simulink model "TVModel_Simulation"  (R2022a)
settings: Solver=FixedStepDiscrete  StartTime=0.0  StopTime=200  FixedStep=0.02  MaxStep=0.01  RelTol=1e-3
undefined symbols (not defined in the file or in its folder): TV
libraries: simulink x5, simulink_extras x3, dspstat3 x2, sharedTrackingLibrary x1, slpidlib x1, eeGeneralControl x1
(part 3 of 4)

== system TVModel_Simulation/Subsystem/Subsystem1/Torque Distribution/MPC/Faults detection/Subsystem2 ==
  In Bus Element : Inport  PortName=dynamics_data  Element=vx
  In Bus Element1 : Inport  Port=2  PortName=driver_inputs  Element=throttle
  OCP Status : Inport  Port=3
  Constant : Constant  Value=3
  Constant1 : Constant  Value=TV.MPC.N/TV.MPC.T*0.1-1
  Constant2 : Constant  Value=TV.LV.TORQUE.T_peak_motor*[0.3;0.3;1;1]
  Discrete FIR Filter : DiscreteFir  Coefficients=ones(1,TV.MPC.N/TV.MPC.T*0.1)
  Less Than : RelationalOperator  Operator=<  OutDataTypeStr=boolean  RndMeth=Simplest  InputSameDT=off
  Less Than1 : RelationalOperator  OutDataTypeStr=boolean  RndMeth=Simplest  InputSameDT=off
  OR : Logic  Operator=OR  Inputs=1  IconShape=distinctive  AllPortsSameDT=off  OutDataTypeStr=boolean
  Product : Product
  Simple Torque : Outport
  flag : Outport  Port=2
  wires:
  OCP Status/1 -> Discrete FIR Filter/1
  Less Than1/1 -> ?  "buffer_flag"
  Discrete FIR Filter/1 -> Less Than1/1
  Constant1/1 -> Less Than1/2
  Product/1 -> Simple Torque/1
  In Bus Element1/1 -> Product/1
  Constant2/1 -> Product/2
  Less Than/1 -> OR/1, flag/1
  In Bus Element/1 -> Less Than/1  "vx"
  Constant/1 -> Less Than/2

== system TVModel_Simulation/Subsystem/Subsystem1/Torque Distribution/MPC/Polytopic Constraints/Accelerator mapping  ==
  acc : Inport
  Constant : Constant
  Divide : Product  Inputs=*/
  Divide1 : Product  Inputs=/*
  Exponent < 0 : Constant  Value=-1.5
  Power : Math  Operator=pow
  Subtract : Sum  Inputs=-+
  Sum : Sum  Inputs=|++
  mapped acc : Outport
  Out Bus Element1 : Outport  Port=2  PortName=TV_Info  Element=acc_map
  wires:
  acc/1 -> Subtract/1, Divide/1
  Subtract/1 -> Divide/2
  Constant/1 -> Sum/2, Divide1/2, Subtract/2
  Divide/1 -> Power/1
  Exponent < 0/1 -> Power/2
  Power/1 -> Sum/1
  Sum/1 -> Divide1/1
  Divide1/1 -> Out Bus Element1/1, mapped acc/1  "acc_map"

== system TVModel_Simulation/Subsystem/Subsystem1/Torque Distribution/MPC/Polytopic Constraints/Power Limiter ==
  In Bus Element5 : Inport  PortName=hv
  In Bus Element4 : Inport  PortName=hv
  In Bus Element3 : Inport  PortName=hv  Element=Pmax_tractive
  In Bus Element1 : Inport  PortName=hv  Element=current
  In Bus Element2 : Inport  PortName=hv  Element=voltage
  If : If  IfExpression=u1 < 0
  If Action Subsystem : Subsystem  TreatAsAtomicUnit=on
  If Action Subsystem1 : Subsystem  TreatAsAtomicUnit=on
  Merge : Merge
  Product : Product
  Subtract : Sum  Inputs=+-
  Out1 : Outport
  wires:
  In Bus Element1/1 -> Product/1  "hv"
  In Bus Element2/1 -> Product/2  "hv"
  In Bus Element3/1 -> Subtract/1  "hv"
  Product/1 -> Subtract/2
  Subtract/1 -> If Action Subsystem/2(Inport), If/1
  If/1 -> If Action Subsystem/Action
  If/2 -> If Action Subsystem1/Action
  If Action Subsystem1/1(Out1) -> Merge/2
  If Action Subsystem/1(Out1) -> Merge/1
  Merge/1 -> Out1/1
  In Bus Element5/1 -> If Action Subsystem/1(hv)  "hv"
  In Bus Element4/1 -> If Action Subsystem1/1(hv)  "hv"

== system TVModel_Simulation/Subsystem/Subsystem1/Torque Distribution/MPC/Polytropic Matrix/Efficiency limit ==
  Motor_Torque : Inport  OutDataTypeStr=double  PortDimensions=4
  In Bus Element34 : Inport  Port=2  PortName=dynamics_data  Element=omega_wheels
  In Bus Element2 : Inport  Port=2  PortName=dynamics_data  Element=omega_wheels
  "     " : Gain  Gain=TV.LV.inv_efficiency
  "      " : Gain  Gain=1/TV.LV.inv_efficiency
  Constant : Constant
  Divide : Product  Inputs=*/
  Gain2 : Gain  Gain=TV.CAR.Tau
  Power to engines : Subsystem
  Saturation : Saturate  UpperLimit=19900*pi/30  LowerLimit=100*pi/30
  Switch3 : Switch  Criteria=u2 > Threshold  SaturateOnIntegerOverflow=off  InputSameDT=off
  Limit : Outport
  wires:
  Power to engines/1(Efficiency) -> "      "/1, "     "/1
  "      "/1 -> Switch3/3  "Braking"
  "     "/1 -> Switch3/1, Divide/2  "Driving"
  Motor_Torque/1 -> Power to engines/2(Torque)
  In Bus Element34/1 -> Gain2/1
  Gain2/1 -> Saturation/1
  In Bus Element2/1 -> Switch3/2
  Divide/1 -> Limit/1
  Saturation/1 -> Power to engines/1(omega_motor)
  Constant/1 -> Divide/1

== system TVModel_Simulation/Subsystem/Subsystem1/Torque Distribution/MPC/States constraints/Anti reverse wheelspin ==
  lbu_in : Inport
  slip_ratio : Inport  Port=2  PortName=dynamics_data
  Constant : Constant  Value=-0.5
  Less Than : RelationalOperator  OutDataTypeStr=boolean  RndMeth=Simplest  InputSameDT=off
  Product : Product
  lbu_out : Outport
  wires:
  Constant/1 -> Less Than/2
  Less Than/1 -> Product/2
  slip_ratio/1 -> Less Than/1
  lbu_in/1 -> Product/1
  Product/1 -> lbu_out/1  "lbu_out"

== system TVModel_Simulation/Subsystem/Subsystem1/Torque Distribution/MPC/States constraints/Brake & ESP ==
  ubu_in : Inport
  In Bus Element13 : Inport  Port=2  PortName=brake_signal  Element=regen
  Constant : Constant
  Constant1 : Constant  Value=0
  Product : Product
  Switch : Switch  Criteria=u2 > Threshold  Threshold=0.95  SaturateOnIntegerOverflow=off  InputSameDT=off
  ubu_out : Outport
  wires:
  Constant/1 -> Switch/3
  Constant1/1 -> Switch/1
  ubu_in/1 -> Product/1
  Switch/1 -> Product/2
  Product/1 -> ubu_out/1
  In Bus Element13/1 -> Switch/2

== system TVModel_Simulation/Subsystem/Subsystem1/Torque Distribution/MPC/States constraints/Bus lbu ==
  lbu : Inport
  C Function : CFunction  OutputCode=|
      | int i,j;
      | for (i = 0; i < N; i++) {
      |  for (j = 0; j < nu; j++) {
      |   out_x[i*nu+j] = in_x[j];
      |  }
      | }
  Constant1 : Constant  Value=TV.MPC.N-1  OutDataTypeStr=uint8  SampleTime=TV.MPC.T/TV.MPC.N
  Constant3 : Constant  Value=TV.MPC.nu  OutDataTypeStr=uint8  SampleTime=TV.MPC.T/TV.MPC.N
  Out : Outport
  wires:
  Constant1/1 -> C Function/2
  C Function/1 -> Out/1
  Constant3/1 -> C Function/3
  lbu/1 -> C Function/1

== system TVModel_Simulation/Subsystem/Subsystem1/Torque Distribution/MPC/States constraints/Bus ubu ==
  ubu : Inport
  C Function : CFunction  OutputCode=|
      | int i,j;
      | for (i = 0; i < N; i++) {
      |  for (j = 0; j < nu; j++) {
      |   out_x[i*nu+j] = in_x[j];
      |  }
      | }
  Constant1 : Constant  Value=TV.MPC.N-1  OutDataTypeStr=uint8  SampleTime=TV.MPC.T/TV.MPC.N
  Constant3 : Constant  Value=TV.MPC.nu  OutDataTypeStr=uint8  SampleTime=TV.MPC.T/TV.MPC.N
  Out : Outport
  wires:
  Constant1/1 -> C Function/2
  C Function/1 -> Out/1
  Constant3/1 -> C Function/3
  ubu/1 -> C Function/1

== system TVModel_Simulation/Subsystem/Subsystem1/Torque Distribution/MPC/States constraints/Hydraulic brakes ==
  In1 : Inport
  In Bus Element7 : Inport  Port=2  PortName=dynamics_data  Element=brake_torque
  Brake friction : Gain  Commented=on  Gain=0.8
  Braking Areas : Constant  Commented=on  Value=[TV.CAR.BrkArea_front;TV.CAR.BrkArea_front;TV.CAR.BrkArea_rear;TV.CAR.BrkArea_rear]
  Braking Disk Radii : Constant  Commented=on  Value=[TV.CAR.DiskDiameter_front;TV.CAR.DiskDiameter_front;TV.CAR.DiskDiameter_rear;TV.CAR.DiskDiameter_rear]/2
  Product : Product  Commented=on
  Product1 : Product  Commented=on
  Subtract : Sum
  Wheel2Motor : Gain  Gain=1/TV.CAR.Tau
  Out1 : Outport
  wires:
  Brake friction/1 -> Product1/1
  Wheel2Motor/1 -> Subtract/2
  In Bus Element7/1 -> Wheel2Motor/1
  Subtract/1 -> Out1/1
  In1/1 -> Subtract/1
  Braking Areas/1 -> Product/2
  Braking Disk Radii/1 -> Product1/2
  Product/1 -> Brake friction/1

== system TVModel_Simulation/Subsystem/Subsystem1/Torque Distribution/MPC/States constraints/LMUx Correction ==
  LMUx Front : Constant  Value=0.75
  LMUx Rear : Constant  Value=0.75
  Nominal LMUx : Gain  Gain=1/0.93
  Vector Concatenate : Concatenate  NumInputs=4
  Out1 : Outport
  wires:
  LMUx Rear/1 -> Vector Concatenate/4, Vector Concatenate/3
  LMUx Front/1 -> Vector Concatenate/1, Vector Concatenate/2
  Nominal LMUx/1 -> Out1/1
  Vector Concatenate/1 -> Nominal LMUx/1

== system TVModel_Simulation/Subsystem/Subsystem1/Torque Distribution/MPC/States constraints/Load Transfer calculation ==
  In Bus Element : Inport  PortName=dynamics_data
  Fz FL : Subsystem
  Fz FR : Subsystem
  Fz RL : Subsystem
  Fz RR : Subsystem
  Mux : Mux
  Fz [4x1] : Outport
  Out Bus Element4 : Outport  Port=2  PortName=TV_Info  Element=fz_fl
  Out Bus Element1 : Outport  Port=2  PortName=TV_Info  Element=fz_fr
  Out Bus Element2 : Outport  Port=2  PortName=TV_Info  Element=fz_rl
  Out Bus Element3 : Outport  Port=2  PortName=TV_Info  Element=fz_rr
  wires:
  In Bus Element/1 -> Fz FL/1(dynamics_data), Fz FR/1(dynamics_data), Fz RL/1(dynamics_data), Fz RR/1(dynamics_data)
  Fz FL/1(TV_Info) -> Out Bus Element4/1, Mux/1  "Fz_FL"
  Fz FR/1(TV_Info) -> Mux/2, Out Bus Element1/1  "Fz_FR"
  Fz RL/1(TV_Info) -> Out Bus Element2/1, Mux/3  "Fz_RL"
  Fz RR/1(TV_Info) -> Out Bus Element3/1, Mux/4  "Fz_RR"
  Mux/1 -> Fz [4x1]/1

== system TVModel_Simulation/Subsystem/Subsystem1/Torque Distribution/MPC/States constraints/Low YRD ==
  In Bus Element13 : Inport  PortName=brake_signal
  ubu : Inport  Port=2
  YRD : Inport  Port=3
  lbu : Inport  Port=4
  In Bus Element1 : Inport  Port=5  PortName=driver_inputs
  lbu_max : Inport  Port=6
  Demux : Demux
  Demux1 : Demux
  Mux : Mux  Inputs=10
  Mz = 0 Bound logic : Subsystem
  Output : Outport
  wires:
  lbu_max/1 -> Mux/10
  In Bus Element1/1 -> Mz = 0 Bound logic/3(driver_inputs)
  YRD/1 -> Mz = 0 Bound logic/2(YRD)
  In Bus Element13/1 -> Mz = 0 Bound logic/1(brake_signal)
  lbu/1 -> Demux1/1
  Demux1/1 -> Mux/6
  Demux1/4 -> Mux/9
  Demux1/2 -> Mux/7
  Demux1/3 -> Mux/8
  Mz = 0 Bound logic/1(flag) -> Mux/1
  Demux/4 -> Mux/5
  Demux/3 -> Mux/4
  Demux/2 -> Mux/3
  Demux/1 -> Mux/2
  ubu/1 -> Demux/1
  Mux/1 -> Output/1

== system TVModel_Simulation/Subsystem/Subsystem1/Torque Distribution/MPC/States constraints/Slip Angle calculation ==
  In Bus Element{,2..4} (4 alike) : Inport  PortName=dynamics_data
  In Bus Element12 : Inport  Port=2  PortName=front_wheel_angles
  In Bus Element1 : Inport  Port=2  PortName=front_wheel_angles
  Mux : Mux
  Slip Angle FL : Subsystem
  Slip Angle FR : Subsystem
  Slip Angle RL : Subsystem
  Slip Angle RR : Subsystem
  Slip angles [4x1] : Outport
  Out Bus Element4 : Outport  Port=2  PortName=TV_Info  Element=slip_angle_FL
  Out Bus Element1 : Outport  Port=2  PortName=TV_Info  Element=slip_angle_FR
  Out Bus Element2 : Outport  Port=2  PortName=TV_Info  Element=slip_angle_RL
  Out Bus Element3 : Outport  Port=2  PortName=TV_Info  Element=slip_angle_RR
  wires:
  In Bus Element4/1 -> Slip Angle RR/1(dynamics_data)
  In Bus Element3/1 -> Slip Angle RL/1(dynamics_data)
  In Bus Element2/1 -> Slip Angle FR/1(dynamics_data)
  In Bus Element1/1 -> Slip Angle FR/2(front_wheel_angles)
  In Bus Element12/1 -> Slip Angle FL/2(front_wheel_angles)
  In Bus Element/1 -> Slip Angle FL/1(dynamics_data)
  Slip Angle FL/1(TV_Info) -> Mux/1, Out Bus Element4/1  "alpha_FL"
  Slip Angle FR/1(TV_Info) -> Mux/2, Out Bus Element1/1  "alpha_FR"
  Slip Angle RL/1(TV_Info) -> Mux/3, Out Bus Element2/1  "alpha_RL"
  Slip Angle RR/1(TV_Info) -> Out Bus Element3/1, Mux/4  "alpha_RR"
  Mux/1 -> Slip angles [4x1]/1

== system TVModel_Simulation/Subsystem/Subsystem1/Torque Distribution/MPC/States constraints/lbu_dot ==
  In Bus Element13 : Inport  PortName=brake_signal  Element=regen
  Motor_Torque : Inport  Port=2
  YRD : Inport  Port=3
  In Bus Element : Inport  Port=4  PortName=dynamics_data  Element=yaw_rate
  AND : Logic  IconShape=distinctive  AllPortsSameDT=off  OutDataTypeStr=boolean
  Abs : Abs  SaturateOnIntegerOverflow=off
  Constant5 : Constant  Value=5
  Constant6 : Constant  Value=-TV.LV.TORQUE.T_peak_motor
  Constant8 : Constant  Value=100
  Constant9 : Constant  Value=TV.LV.GENERAL.BrakeThresh
  Less Than3 : RelationalOperator  Operator=<  OutDataTypeStr=boolean  RndMeth=Simplest  InputSameDT=off
  Less Than4 : RelationalOperator  Operator=<  OutDataTypeStr=boolean  RndMeth=Simplest  InputSameDT=off
  Product : Product
  Subtract : Sum  Inputs=+-
  Sum : Sum  Inputs=|+-
  Sum1 : Sum  Inputs=|++
  Switch1 : Switch  Criteria=u2 > Threshold  SaturateOnIntegerOverflow=off  InputSameDT=off
  Unit Delay1 : UnitDelay  SampleTime=-1  HasFrameUpgradeWarning=on
  lbu_in : Outport
  wires:
  Less Than4/1 -> AND/2
  Less Than3/1 -> AND/1
  Unit Delay1/1 -> Less Than3/1
  Constant9/1 -> Less Than4/1, Less Than3/2
  In Bus Element13/1 -> Unit Delay1/1, Less Than4/2
  Constant5/1 -> Product/2
  Abs/1 -> Sum1/2
  Product/1 -> Abs/1
  Constant8/1 -> Sum1/1
  YRD/1 -> Subtract/2
  Subtract/1 -> Product/1
  Sum1/1 -> Sum/2
  In Bus Element/1 -> Subtract/1
  Sum/1 -> Switch1/3
  AND/1 -> Switch1/2
  Constant6/1 -> Switch1/1
  Switch1/1 -> lbu_in/1
  Motor_Torque/1 -> Sum/1

== system TVModel_Simulation/Subsystem/Subsystem1/Torque Distribution/MPC/States constraints/ubu_dot ==
  Motor_Torque : Inport
  YRD : Inport  Port=2
  In Bus Element : Inport  Port=3  PortName=dynamics_data  Element=yaw_rate
  Abs : Abs  SaturateOnIntegerOverflow=off
  Constant6 : Constant  Value=5
  Constant7 : Constant  Value=100
  Product : Product
  Subtract : Sum  Inputs=+-
  Sum : Sum  Inputs=|++
  Sum1 : Sum  Inputs=|++
  Output : Outport
  wires:
  Sum/1 -> Output/1
  YRD/1 -> Subtract/2
  In Bus Element/1 -> Subtract/1
  Subtract/1 -> Product/1
  Constant6/1 -> Product/2
  Product/1 -> Abs/1
  Constant7/1 -> Sum1/1
  Abs/1 -> Sum1/2
  Sum1/1 -> Sum/2
  Motor_Torque/1 -> Sum/1

== system TVModel_Simulation/Subsystem/Subsystem1/Torque Distribution/MPC/Weights generation/Efficiency limit ==
  Motor_Torque : Inport  OutDataTypeStr=double  PortDimensions=4
  In Bus Element34 : Inport  Port=2  PortName=dynamics_data  Element=omega_wheels
  In Bus Element2 : Inport  Port=2  PortName=dynamics_data  Element=omega_wheels
  "     " : Gain  Gain=TV.LV.inv_efficiency
  "      " : Gain  Gain=1/TV.LV.inv_efficiency
  Constant : Constant
  Divide : Product  Inputs=*/
  Gain2 : Gain  Gain=TV.CAR.Tau
  MATLAB Function : MATLAB Function  TreatAsAtomicUnit=on
  Power to engines : Subsystem
  Saturation : Saturate  UpperLimit=19900*pi/30  LowerLimit=100*pi/30
  Switch3 : Switch  Criteria=u2 > Threshold  SaturateOnIntegerOverflow=off  InputSameDT=off
  Limit : Outport
  wires:
  Power to engines/1(Efficiency) -> "      "/1, "     "/1
  "      "/1 -> Switch3/3  "Braking"
  "     "/1 -> Switch3/1, Divide/2  "Driving"
  Motor_Torque/1 -> MATLAB Function/2(T), Power to engines/2(Torque)
  In Bus Element34/1 -> Gain2/1
  Gain2/1 -> Saturation/1
  In Bus Element2/1 -> Switch3/2
  MATLAB Function/1(u) -> Limit/1
  Saturation/1 -> Power to engines/1(omega_motor)
  Divide/1 -> MATLAB Function/1("u ")
  Constant/1 -> Divide/1

== system TVModel_Simulation/Subsystem/Subsystem1/Torque Distribution/MPC/Weights generation/Subsystem1 ==
  front_wheel_angles : Inport
  Steer Activation : Subsystem
  epsilon : Outport
  wires:
  front_wheel_angles/1 -> Steer Activation/1(front_wheel_angle)  "delta"
  Steer Activation/1(epsilon) -> epsilon/1

== system TVModel_Simulation/Subsystem/Subsystem1/Torque Distribution/MPC/ States/Extended Kalman Filter/ Parameter Bus  ==
  Motor_Torque : Inport
  In Bus Element1 : Inport  Port=2  PortName=slip_ratio  Element=fl
  In Bus Element2 : Inport  Port=2  PortName=slip_ratio  Element=fr
  In Bus Element3 : Inport  Port=2  PortName=slip_ratio  Element=rl
  In Bus Element4 : Inport  Port=2  PortName=slip_ratio  Element=rr
  In Bus Element11 : Inport  Port=3  PortName=front_wheel_angles  Element=single_axis
  Demux1 : Demux
  Mux : Mux  Inputs=9
  Signal Specification{4..7} (4 alike) : SignalSpecification  Dimensions=1
  p : Outport
  wires:
  In Bus Element4/1 -> Mux/5  "slip_ratio_rr"
  In Bus Element3/1 -> Mux/4  "slip_ratio_rl"
  In Bus Element2/1 -> Mux/3  "slip_ratio_fr"
  In Bus Element1/1 -> Mux/2  "slip_ratio_fl"
  Mux/1 -> p/1
  Motor_Torque/1 -> Demux1/1
  In Bus Element11/1 -> Mux/1  "delta"
  Demux1/1 -> Signal Specification4/1
  Demux1/2 -> Signal Specification5/1
  Demux1/3 -> Signal Specification6/1
  Demux1/4 -> Signal Specification7/1
  Signal Specification4/1 -> Mux/6
  Signal Specification5/1 -> Mux/7
  Signal Specification6/1 -> Mux/8
  Signal Specification7/1 -> Mux/9

== system TVModel_Simulation/Subsystem/Subsystem1/Torque Distribution/MPC/ States/Extended Kalman Filter/measurement_kalman_simulink ==
  measurement_kalman_simulink : TriggerPort  TriggerType=function-call  IsSimulinkFunction=on  FunctionName=measurement_kalman_simulink  VariantControl=(inherit)
  h(x) : MATLAB Function  TreatAsAtomicUnit=on
  x : ArgIn  DisableCoverage=on  OutDataTypeStr=single  PortDimensions=4  ArgumentName=x
  y : ArgOut  DisableCoverage=on  OutDataTypeStr=single  ArgumentName=y
  wires:
  x/1 -> h(x)/1(x)
  h(x)/1(y) -> y/1

== system TVModel_Simulation/Subsystem/Subsystem1/Torque Distribution/MPC/ States/Extended Kalman Filter/state_update_kalman_simulink ==
  Parameters : Inport
  state_update_kalman_simulink : TriggerPort  TriggerType=function-call  IsSimulinkFunction=on  FunctionName=state_update_kalman_simulink  VariantControl=(inherit)
  f(x,u) : MATLAB Function  TreatAsAtomicUnit=on
  x : ArgIn  DisableCoverage=on  OutDataTypeStr=single  PortDimensions=4  ArgumentName=x
  xout : ArgOut  DisableCoverage=on  OutDataTypeStr=single  PortDimensions=4  ArgumentName=xout
  wires:
  f(x,u)/1(xout) -> xout/1
  x/1 -> f(x,u)/1(x)
  Parameters/1 -> f(x,u)/2(u)

== system TVModel_Simulation/Subsystem/Subsystem1/Torque Distribution/MPC/ States/Yrd 0 When Steering 0/Steer Limit ==
  front_wheel_angle : Inport
  Inport : Inport  Port=2
  Constant : Constant  Value=3.5*pi/180
  Constant1 : Constant  Value=pi/180/4
  Data Type Conversion : DataTypeConversion  OutDataTypeStr=double  SaturateOnIntegerOverflow=off  RndMeth=Floor
  Less Than : RelationalOperator  OutDataTypeStr=boolean  RndMeth=Simplest  InputSameDT=off
  Less Than1 : RelationalOperator  OutDataTypeStr=boolean  RndMeth=Simplest  InputSameDT=off
  Product : Product
  Product1 : Product
  S-R Flip-Flop : simulink_extras/Flip Flops/S-R Flip-Flop  initial_condition=0
  Saturation : Saturate  UpperLimit=2  LowerLimit=1
  Terminator : Terminator
  Transfer Fcn : TransferFcn  Denominator=[1/(2*pi*2) 1]
  vx_normalization : Gain  Gain=1/20
  steer_limit : Outport
  wires:
  S-R Flip-Flop/2 -> Terminator/1
  S-R Flip-Flop/1 -> Data Type Conversion/1
  Less Than/1 -> S-R Flip-Flop/1
  Less Than1/1 -> S-R Flip-Flop/2
  Inport/1 -> vx_normalization/1
  vx_normalization/1 -> Saturation/1
  Saturation/1 -> Product/1, Product1/2
  front_wheel_angle/1 -> Less Than/1, Less Than1/2
  Product/1 -> Less Than1/1
  Constant1/1 -> Product/2
  Product1/1 -> Less Than/2
  Constant/1 -> Product1/1
  Data Type Conversion/1 -> Transfer Fcn/1  "flip_flop"
  Transfer Fcn/1 -> steer_limit/1

== system TVModel_Simulation/Subsystem/Subsystem1/Torque Distribution/MPC/Faults detection/Power flag/Efficiency limit ==
  Motor_Torque : Inport  OutDataTypeStr=double  PortDimensions=4
  In Bus Element34 : Inport  Port=2  PortName=dynamics_data  Element=omega_wheels
  Divide2 : Product  Inputs=*/*
  Gain2 : Gain  Gain=TV.CAR.Tau
  Power to engines : Subsystem
  Saturation : Saturate  UpperLimit=19900*pi/30  LowerLimit=100*pi/30
  Limit : Outport
  wires:
  Divide2/1 -> Limit/1  "Limit"
  Saturation/1 -> Power to engines/1(omega_motor), Divide2/1
  Gain2/1 -> Saturation/1
  In Bus Element34/1 -> Gain2/1
  Motor_Torque/1 -> Power to engines/2(Torque), Divide2/3
  Power to engines/1(Efficiency) -> Divide2/2

== system TVModel_Simulation/Subsystem/Subsystem1/Torque Distribution/MPC/Polytopic Constraints/Power Limiter/If Action Subsystem ==
  In Bus Element5 : Inport  PortName=hv  Element=Pmax_tractive
  Inport : Inport  Port=2
  Action Port : ActionPort
  Discrete PID Controller : slpidlib/PID Controller  Controller=PI  Form=Parallel  TimeDomain=Discrete-time  UseExternalTs=on  SampleTime=-1  IntegratorMethod=Forward Euler  FilterMethod=Forward Euler  ControllerParametersSource=internal  P=1e-3  I=0  UseKiTs=off  D=0  N=100  UseFilter=on  TunerSelectOption=Transfer Function Based (PID Tuner App)  InitialConditionSource=internal  InitialConditionForIntegrator=0  InitialConditionForFilter=0  DifferentiatorICPrevScaledInput=0  ExternalReset=none  TrackingMode=off  Kt=1  LimitOutput=off  SatLimitsSource=internal  UpperSaturationLimit=inf  LowerSaturationLimit=-inf  LinearizeAsGain=off  AntiWindupMode=none  Kb=1  POutMin=[]  POutMax=[]  IOutMin=[]  IOutMax=[]  DOutMin=[]  DOutMax=[]  NOutMin=[]  NOutMax=[]  SumOutMin=[]  SumOutMax=[]  SaturationOutMin=[]  SaturationOutMax=[]  PParamMin=[]  PParamMax=[]  IParamMin=[]  IParamMax=[]  DParamMin=[]  DParamMax=[]  NParamMin=[]  NParamMax=[]  KbParamMin=[]  KbParamMax=[]  KtParamMin=[]  KtParamMax=[]  KbOutMin=[]  KbOutMax=[]  KtOutMin=[]  KtOutMax=[]  IntegratorOutMin=[]  IntegratorOutMax=[]  FilterOutMin=[]  FilterOutMax=[]  SumI1OutMin=[]  SumI1OutMax=[]  SumI2OutMin=[]  SumI2OutMax=[]  SumI3OutMin=[]  SumI3OutMax=[]  SumI4OutMin=[]  SumI4OutMax=[]  SumDOutMin=[]  SumDOutMax=[]  DifferentiatorOutMin=[]  DifferentiatorOutMax=[]  FilterDiffOutCoefMin=[]  FilterDiffOutCoefMax=[]  ReciprocalOutMin=[]  ReciprocalOutMax=[]  SumDenOutMin=[]  SumDenOutMax=[]  SumNumOutMin=[]  SumNumOutMax=[]  DivideOutMin=[]  DivideOutMax=[]  UdiffTsProdOutMin=[]  UdiffTsProdOutMax=[]  NTsProdOutMin=[]  NTsProdOutMax=[]  UintegralTsProdOutMin=[]  UintegralTsProdOutMax=[]  UngainTsProdOutMin=[]  UngainTsProdOutMax=[]  IntegratorContinuousStateAttributes=''  IntegratorStateMustResolveToSignalObject=off  IntegratorRTWStateStorageClass=Auto  FilterContinuousStateAttributes=''  FilterStateMustResolveToSignalObject=off  FilterRTWStateStorageClass=Auto  ParallelPVariant=InternalParameters  IdealPVariant=Disabled  IVariant=InternalParameters  DVariant=Disabled  IntegratorVariant=Discrete  SatVariant=Disabled  AWVariant=Passthrough  PCopyVariant=Disabled  TRVariant=Disabled  FdbkBlocksVariant=Forward  IdealPFdbkVariant=Disabled  SatFdbkVariant=Disabled  DerivativeFilterVariant=Disabled  NVariant=Disabled  NCopyVariant=Disabled_SignalSpec  FilterICVariant=Disabled  IntegratorICVariant=InternalICs  ExternalResetVariant=Disabled  TRSumVariant=Passthrough  SumFdbkVariant=Disabled  SumVariant=Sum_PI  TsampFilterVariant=InternalTs  TsampNgainVariant=Passthrough  TsampIntegralVariant=ExternalTs  ExternalSaturationOutDataTypeStr=Inherit: Same as second input  aMode=0
  Saturation : Saturate  UpperLimit=inf  LowerLimit=0
  Sum : Sum
  Out1 : Outport
  wires:
  Sum/1 -> Saturation/1
  Discrete PID Controller/1 -> Sum/2  "PID_output"
  Inport/1 -> Discrete PID Controller/1
  In Bus Element5/1 -> Sum/1  "hv"
  Saturation/1 -> Out1/1

== system TVModel_Simulation/Subsystem/Subsystem1/Torque Distribution/MPC/Polytopic Constraints/Power Limiter/If Action Subsystem1 ==
  In Bus Element5 : Inport  PortName=hv  Element=Pmax_tractive
  Action Port : ActionPort
  Out1 : Outport
  wires:
  In Bus Element5/1 -> Out1/1

== system TVModel_Simulation/Subsystem/Subsystem1/Torque Distribution/MPC/Polytropic Matrix/Efficiency limit/Power to engines ==
  omega_motor : Inport
  Torque : Inport  Port=2
  2-D Lookup Table : Lookup_n-D  BreakpointsForDimension1=TV.LV.efficiency_LUT.Omega  BreakpointsForDimension2=TV.LV.efficiency_LUT.Torque  Table=TV.LV.efficiency_LUT.Eta  InternalRulePriority=Speed  RndMeth=Simplest
      settings: InputPortMap=u0,u1
  Abs : Abs  SaturateOnIntegerOverflow=off
  Saturation : Saturate  UpperLimit=1  LowerLimit=0.3
  Efficiency : Outport
  wires:
  Torque/1 -> Abs/1
  2-D Lookup Table/1 -> Saturation/1
  Saturation/1 -> Efficiency/1  "Efficiency"
  omega_motor/1 -> 2-D Lookup Table/1  "[rad/s]"
  Abs/1 -> 2-D Lookup Table/2

== system TVModel_Simulation/Subsystem/Subsystem1/Torque Distribution/MPC/States constraints/Load Transfer calculation/Fz FL ==
  In Bus Element : Inport  PortName=dynamics_data  Element=ay
  In Bus Element1 : Inport  PortName=dynamics_data  Element=vx
  In Bus Element2 : Inport  PortName=dynamics_data  Element=ax
  Drag moment : Gain  Gain=0.5*TV.CAR.rho*TV.CAR.CdA*TV.CAR.hcop/TV.CAR.wb*0.5
  Lateral Load Transfer : Gain  Gain=TV.CAR.m/TV.CAR.tf*TV.CAR.hcog*0.5*0.5
  Lift Force : Gain  Gain=0.5*TV.CAR.rho*TV.CAR.ClA*(1-TV.CAR.xcop/TV.CAR.wb)*0.5
  Longitudinal Load Transfer : Gain  Gain=TV.CAR.m/TV.CAR.wb*TV.CAR.hcog*0.5
  Square1 : Math  Operator=square
  Square2 : Math  Operator=square
  Static Load Front : Constant  Value=TV.CAR.Fzf
  Subtract : Sum  Inputs=+++-+
  Unary Minus : UnaryMinus
  Unary Minus1 : UnaryMinus
  TV_Info : Outport
  wires:
  Lift Force/1 -> Subtract/3
  In Bus Element1/1 -> Square1/1, Square2/1
  Square2/1 -> Drag moment/1
  In Bus Element2/1 -> Unary Minus1/1
  Longitudinal Load Transfer/1 -> Subtract/5
  Lateral Load Transfer/1 -> Subtract/2
  Square1/1 -> Lift Force/1
  Static Load Front/1 -> Subtract/1
  Drag moment/1 -> Subtract/4
  Subtract/1 -> TV_Info/1
  In Bus Element/1 -> Unary Minus/1
  Unary Minus/1 -> Lateral Load Transfer/1
  Unary Minus1/1 -> Longitudinal Load Transfer/1

== system TVModel_Simulation/Subsystem/Subsystem1/Torque Distribution/MPC/States constraints/Load Transfer calculation/Fz FR ==
  In Bus Element : Inport  PortName=dynamics_data  Element=ay
  In Bus Element1 : Inport  PortName=dynamics_data  Element=vx
  In Bus Element2 : Inport  PortName=dynamics_data  Element=ax
  Drag moment : Gain  Gain=0.5*TV.CAR.rho*TV.CAR.CdA*TV.CAR.hcop/TV.CAR.wb*0.5
  Lateral Load Transfer : Gain  Gain=TV.CAR.m/TV.CAR.tf*TV.CAR.hcog*0.5*0.5
  Lift Force : Gain  Gain=0.5*TV.CAR.rho*TV.CAR.ClA*(1 - TV.CAR.xcop/TV.CAR.wb)*0.5
  Longitudinal Load Transfer : Gain  Gain=TV.CAR.m/TV.CAR.wb*TV.CAR.hcog*0.5
  Square1 : Math  Operator=square
  Square2 : Math  Operator=square
  Static Load Front : Constant  Value=TV.CAR.Fzf
  Subtract : Sum  Inputs=+-+-+
  Unary Minus : UnaryMinus
  Unary Minus1 : UnaryMinus
  TV_Info : Outport
  wires:
  Square2/1 -> Drag moment/1
  Lift Force/1 -> Subtract/3
  In Bus Element2/1 -> Unary Minus1/1
  Longitudinal Load Transfer/1 -> Subtract/5
  Lateral Load Transfer/1 -> Subtract/2
  Square1/1 -> Lift Force/1
  Static Load Front/1 -> Subtract/1
  In Bus Element1/1 -> Square2/1, Square1/1
  In Bus Element/1 -> Unary Minus/1
  Drag moment/1 -> Subtract/4
  Subtract/1 -> TV_Info/1
  Unary Minus/1 -> Lateral Load Transfer/1
  Unary Minus1/1 -> Longitudinal Load Transfer/1

== system TVModel_Simulation/Subsystem/Subsystem1/Torque Distribution/MPC/States constraints/Load Transfer calculation/Fz RL ==
  In Bus Element : Inport  PortName=dynamics_data  Element=ay
  In Bus Element1 : Inport  PortName=dynamics_data  Element=vx
  In Bus Element2 : Inport  PortName=dynamics_data  Element=ax
  Drag moment : Gain  Gain=0.5*TV.CAR.rho*TV.CAR.CdA*TV.CAR.hcop/TV.CAR.wb*0.5
  Lateral Load Transfer : Gain  Gain=TV.CAR.m/TV.CAR.tr*TV.CAR.hcog*0.5*0.5
  Lift Force : Gain  Gain=0.5*TV.CAR.rho*TV.CAR.ClA*(TV.CAR.xcop/TV.CAR.wb)*0.5
  Longitudinal Load Transfer : Gain  Gain=TV.CAR.m/TV.CAR.wb*TV.CAR.hcog*0.5
  Square1 : Math  Operator=square
  Square2 : Math  Operator=square
  Static Load Front : Constant  Value=TV.CAR.Fzr
  Subtract : Sum  Inputs=++++-
  Unary Minus : UnaryMinus
  Unary Minus1 : UnaryMinus
  TV_Info : Outport
  wires:
  In Bus Element1/1 -> Square1/1, Square2/1
  Square2/1 -> Drag moment/1
  Lift Force/1 -> Subtract/3
  In Bus Element2/1 -> Unary Minus1/1
  Longitudinal Load Transfer/1 -> Subtract/5
  Lateral Load Transfer/1 -> Subtract/2
  Square1/1 -> Lift Force/1
  Static Load Front/1 -> Subtract/1
  In Bus Element/1 -> Unary Minus/1
  Drag moment/1 -> Subtract/4
  Subtract/1 -> TV_Info/1
  Unary Minus/1 -> Lateral Load Transfer/1
  Unary Minus1/1 -> Longitudinal Load Transfer/1

== system TVModel_Simulation/Subsystem/Subsystem1/Torque Distribution/MPC/States constraints/Load Transfer calculation/Fz RR ==
  In Bus Element : Inport  PortName=dynamics_data  Element=ay
  In Bus Element1 : Inport  PortName=dynamics_data  Element=vx
  In Bus Element2 : Inport  PortName=dynamics_data  Element=ax
  Drag moment : Gain  Gain=0.5*TV.CAR.rho*TV.CAR.CdA*TV.CAR.hcop/TV.CAR.wb*0.5
  Lateral Load Transfer : Gain  Gain=TV.CAR.m/TV.CAR.tr*TV.CAR.hcog*0.5*0.5
  Lift Force : Gain  Gain=0.5*TV.CAR.rho*TV.CAR.ClA*(TV.CAR.xcop/TV.CAR.wb)*0.5
  Longitudinal Load Transfer : Gain  Gain=TV.CAR.m/TV.CAR.wb*TV.CAR.hcog*0.5
  Square1 : Math  Operator=square
  Square2 : Math  Operator=square
  Static Load Front : Constant  Value=TV.CAR.Fzr
  Subtract : Sum  Inputs=+-++-
  Unary Minus : UnaryMinus
  Unary Minus1 : UnaryMinus
  TV_Info : Outport
  wires:
  Square2/1 -> Drag moment/1
  Lift Force/1 -> Subtract/3
  In Bus Element2/1 -> Unary Minus1/1
  Longitudinal Load Transfer/1 -> Subtract/5
  Lateral Load Transfer/1 -> Subtract/2
  Square1/1 -> Lift Force/1
  Static Load Front/1 -> Subtract/1
  In Bus Element1/1 -> Square2/1, Square1/1
  In Bus Element/1 -> Unary Minus/1
  Drag moment/1 -> Subtract/4
  Subtract/1 -> TV_Info/1
  Unary Minus/1 -> Lateral Load Transfer/1
  Unary Minus1/1 -> Longitudinal Load Transfer/1

== system TVModel_Simulation/Subsystem/Subsystem1/Torque Distribution/MPC/States constraints/Low YRD/Mz = 0 Bound logic ==
  In Bus Element13 : Inport  PortName=brake_signal  Element=regen
  YRD : Inport  Port=2
  In Bus Element1 : Inport  Port=3  PortName=driver_inputs  Element=throttle
  " " : Constant  Value=0.95
  "  " : Constant  Value=TV.LV.GENERAL.ThrottleThresh
  "             " : Constant  Value=TV.LV.GENERAL.YRDTresh
  AND : Logic  IconShape=distinctive  AllPortsSameDT=off  OutDataTypeStr=boolean
  AND1 : Logic  IconShape=distinctive  AllPortsSameDT=off  OutDataTypeStr=boolean
  AND2 : Logic  IconShape=distinctive  AllPortsSameDT=off  OutDataTypeStr=boolean
  Abs : Abs  SaturateOnIntegerOverflow=off
  Constant : Constant  Value=TV.LV.GENERAL.BrakeThresh
  Constant1 : Constant  Value=10
  Data Type Conversion : DataTypeConversion  OutDataTypeStr=double  SaturateOnIntegerOverflow=off  RndMeth=Floor
  Data Type Conversion1 : DataTypeConversion  OutDataTypeStr=double  SaturateOnIntegerOverflow=off  RndMeth=Floor
  Discrete FIR Filter : DiscreteFir  Coefficients=ones(1,TV.MPC.N/TV.MPC.T*0.2)
  Gain : Gain  Gain=2
  Less Than : RelationalOperator  Operator=<=  OutDataTypeStr=fixdt(1,16)  RndMeth=Simplest  InputSameDT=off
  Less Than1 : RelationalOperator  OutDataTypeStr=boolean  RndMeth=Simplest  InputSameDT=off
  Less Than2 : RelationalOperator  Operator=<  OutDataTypeStr=boolean  RndMeth=Simplest  InputSameDT=off
  Less Than3 : RelationalOperator  Operator=<  OutDataTypeStr=boolean  RndMeth=Simplest  InputSameDT=off
  Less Than4 : RelationalOperator  OutDataTypeStr=boolean  RndMeth=Simplest  InputSameDT=off
  Sum : Sum
  flag : Outport
  wires:
  Constant/1 -> Less Than3/1
  Less Than3/1 -> AND2/2
  Less Than2/1 -> AND2/1
  AND2/1 -> AND1/1
  Data Type Conversion1/1 -> Gain/1
  Data Type Conversion/1 -> Sum/2
  Sum/1 -> flag/1
  AND/1 -> Data Type Conversion/1
  Gain/1 -> Sum/1
  AND1/1 -> Data Type Conversion1/1
  " "/1 -> Less Than2/2
  In Bus Element13/1 -> Less Than2/1, Less Than3/2
  Less Than1/1 -> AND/2
  In Bus Element1/1 -> Less Than1/1
  YRD/1 -> Abs/1
  Abs/1 -> Less Than/1
  "             "/1 -> Less Than/2
  "  "/1 -> Less Than1/2
  Discrete FIR Filter/1 -> Less Than4/1
  Less Than4/1 -> AND1/2, AND/1
  Constant1/1 -> Less Than4/2
  Less Than/1 -> Discrete FIR Filter/1

== system TVModel_Simulation/Subsystem/Subsystem1/Torque Distribution/MPC/States constraints/Slip Angle calculation/Slip Angle FL ==
  In Bus Element : Inport  PortName=dynamics_data  Element=vy
  In Bus Element1 : Inport  PortName=dynamics_data  Element=vx
  In Bus Element2 : Inport  PortName=dynamics_data  Element=yaw_rate
  In Bus Element3 : Inport  PortName=dynamics_data  Element=yaw_rate
  In Bus Element12 : Inport  Port=2  PortName=front_wheel_angles  Element=different_axis
  Atan : Trigonometry  Operator=atan2
  Gain : Gain  Gain=TV.CAR.a
  Gain1 : Gain  Gain=TV.CAR.tf/2
  Selector : Selector  InputPortWidth=2  IndexOptions=Index vector (dialog)  Indices=[1]  OutputSizes=1
  Subtract : Sum  Inputs=+-
  Subtract1 : Sum
  Subtract2 : Sum  Inputs=+-
  TV_Info : Outport
  wires:
  In Bus Element12/1 -> Selector/1
  In Bus Element/1 -> Subtract1/1
  Atan/1 -> Subtract2/1
  Subtract1/1 -> Atan/1
  Subtract2/1 -> TV_Info/1
  In Bus Element2/1 -> Gain/1
  Gain1/1 -> Subtract/2
  In Bus Element3/1 -> Gain1/1
  Gain/1 -> Subtract1/2
  Subtract/1 -> Atan/2
  In Bus Element1/1 -> Subtract/1
  Selector/1 -> Subtract2/2

== system TVModel_Simulation/Subsystem/Subsystem1/Torque Distribution/MPC/States constraints/Slip Angle calculation/Slip Angle FR ==
  In Bus Element : Inport  PortName=dynamics_data  Element=vy
  In Bus Element1 : Inport  PortName=dynamics_data  Element=vx
  In Bus Element2 : Inport  PortName=dynamics_data  Element=yaw_rate
  In Bus Element3 : Inport  PortName=dynamics_data  Element=yaw_rate
  In Bus Element12 : Inport  Port=2  PortName=front_wheel_angles  Element=different_axis
  Atan : Trigonometry  Operator=atan2
  Gain : Gain  Gain=TV.CAR.a
  Gain1 : Gain  Gain=TV.CAR.tf/2
  Selector : Selector  InputPortWidth=2  IndexOptions=Index vector (dialog)  Indices=[2]  OutputSizes=1
  Subtract : Sum
  Subtract1 : Sum
  Subtract2 : Sum  Inputs=+-
  TV_Info : Outport
  wires:
  In Bus Element12/1 -> Selector/1
  In Bus Element3/1 -> Gain1/1
  In Bus Element1/1 -> Subtract/1
  In Bus Element2/1 -> Gain/1
  In Bus Element/1 -> Subtract1/1
  Atan/1 -> Subtract2/1
  Subtract1/1 -> Atan/1
  Subtract2/1 -> TV_Info/1
  Gain1/1 -> Subtract/2
  Selector/1 -> Subtract2/2
  Gain/1 -> Subtract1/2
  Subtract/1 -> Atan/2

== system TVModel_Simulation/Subsystem/Subsystem1/Torque Distribution/MPC/States constraints/Slip Angle calculation/Slip Angle RL ==
  In Bus Element : Inport  PortName=dynamics_data  Element=vy
  In Bus Element1 : Inport  PortName=dynamics_data  Element=vx
  In Bus Element2 : Inport  PortName=dynamics_data  Element=yaw_rate
  In Bus Element3 : Inport  PortName=dynamics_data  Element=yaw_rate
  Atan : Trigonometry  Operator=atan2
  Gain : Gain  Gain=TV.CAR.b
  Gain1 : Gain  Gain=TV.CAR.tr/2
  Subtract : Sum  Inputs=+-
  Subtract1 : Sum  Inputs=+-
  TV_Info : Outport
  wires:
  In Bus Element2/1 -> Gain/1
  In Bus Element/1 -> Subtract1/1
  In Bus Element3/1 -> Gain1/1
  In Bus Element1/1 -> Subtract/1
  Subtract1/1 -> Atan/1
  Atan/1 -> TV_Info/1
  Gain1/1 -> Subtract/2
  Gain/1 -> Subtract1/2
  Subtract/1 -> Atan/2

== system TVModel_Simulation/Subsystem/Subsystem1/Torque Distribution/MPC/States constraints/Slip Angle calculation/Slip Angle RR ==
  In Bus Element : Inport  PortName=dynamics_data  Element=vy
  In Bus Element1 : Inport  PortName=dynamics_data  Element=vx
  In Bus Element2 : Inport  PortName=dynamics_data  Element=yaw_rate
  In Bus Element4 : Inport  PortName=dynamics_data  Element=yaw_rate
  Atan : Trigonometry  Operator=atan2
  Gain : Gain  Gain=TV.CAR.b
  Gain1 : Gain  Gain=TV.CAR.tr/2
  Subtract : Sum
  Subtract1 : Sum  Inputs=+-
  TV_Info : Outport
  wires:
  In Bus Element4/1 -> Gain/1
  In Bus Element/1 -> Subtract1/1
  In Bus Element2/1 -> Gain1/1
  In Bus Element1/1 -> Subtract/1
  Subtract1/1 -> Atan/1
  Atan/1 -> TV_Info/1
  Gain1/1 -> Subtract/2
  Gain/1 -> Subtract1/2
  Subtract/1 -> Atan/2

== system TVModel_Simulation/Subsystem/Subsystem1/Torque Distribution/MPC/Weights generation/Efficiency limit/Power to engines ==
  omega_motor : Inport
  Torque : Inport  Port=2
  2-D Lookup Table : Lookup_n-D  BreakpointsForDimension1=TV.LV.efficiency_LUT.Omega  BreakpointsForDimension2=TV.LV.efficiency_LUT.Torque  Table=TV.LV.efficiency_LUT.Eta  InternalRulePriority=Speed  RndMeth=Simplest
      settings: InputPortMap=u0,u1
  Abs : Abs  SaturateOnIntegerOverflow=off
  Saturation : Saturate  UpperLimit=1  LowerLimit=0.3
  Efficiency : Outport
  wires:
  Torque/1 -> Abs/1
  2-D Lookup Table/1 -> Saturation/1
  Saturation/1 -> Efficiency/1  "Efficiency"
  omega_motor/1 -> 2-D Lookup Table/1  "[rad/s]"
  Abs/1 -> 2-D Lookup Table/2

== system TVModel_Simulation/Subsystem/Subsystem1/Torque Distribution/MPC/Weights generation/Subsystem1/Steer Activation ==
  front_wheel_angle : Inport
  AND : Logic  IconShape=distinctive  AllPortsSameDT=off  OutDataTypeStr=boolean
  Abs : Abs  SaturateOnIntegerOverflow=off
  Constant1 : Constant  Value=pi/180
  Constant4 : Constant  Value=pi/180/4
  Delay : Delay  DelayLength=5
  First Activation : Subsystem
  If : If  IfExpression=u1 == 1
  If Action Subsystem : Subsystem  TreatAsAtomicUnit=on
  If Action Subsystem1 : Subsystem  TreatAsAtomicUnit=on
  Less Than : RelationalOperator  Operator=<=  OutDataTypeStr=boolean  RndMeth=Simplest  InputSameDT=off
  Less Than2 : RelationalOperator  Operator=<  OutDataTypeStr=boolean  RndMeth=Simplest  InputSameDT=off
  Merge : Merge
  Moving Average : dspstat3/Moving Average  Method=Sliding window  ForgettingFactorPort=off  SpecifyWindowLength=on  WindowLength=25  ForgettingFactor=0.9  SimulateUsing=Code generation
  S-R Flip-Flop : simulink_extras/Flip Flops/S-R Flip-Flop  initial_condition=0
  Terminator : Terminator
  epsilon : Outport
  wires:
  Constant4/1 -> Less Than2/2
  Moving Average/1 -> Less Than2/1
  Delay/1 -> AND/2
  Less Than/1 -> S-R Flip-Flop/1  "set"
  AND/1 -> S-R Flip-Flop/2  "reset"
  Less Than2/1 -> AND/1  "reset"
  S-R Flip-Flop/2 -> Terminator/1
  Constant1/1 -> Less Than/1
  Merge/1 -> epsilon/1
  front_wheel_angle/1 -> Abs/1
  If/2 -> If Action Subsystem/Action
  S-R Flip-Flop/1 -> First Activation/1(In1), If Action Subsystem/1(Inport), Delay/1  "Q"
  First Activation/1(Out1) -> If/1  "u1"
  If Action Subsystem1/1(epsilon) -> Merge/1
  If Action Subsystem/1(Epsilon) -> Merge/2
  If/1 -> If Action Subsystem1/Action
  Abs/1 -> If Action Subsystem1/1(Inport), Less Than/2, Moving Average/1

== system TVModel_Simulation/Subsystem/Subsystem1/Torque Distribution/MPC/Faults detection/Power flag/Efficiency limit/Power to engines ==
  omega_motor : Inport
  Torque : Inport  Port=2
  2-D Lookup Table : Lookup_n-D  BreakpointsForDimension1=TV.LV.efficiency_LUT.Omega  BreakpointsForDimension2=TV.LV.efficiency_LUT.Torque  Table=TV.LV.efficiency_LUT.Eta  InternalRulePriority=Speed  RndMeth=Simplest
      settings: InputPortMap=u0,u1
  Abs : Abs  SaturateOnIntegerOverflow=off
  Saturation : Saturate  UpperLimit=1  LowerLimit=0.3
  Efficiency : Outport
  wires:
  Abs/1 -> 2-D Lookup Table/2
  omega_motor/1 -> 2-D Lookup Table/1  "[rad/s]"
  Saturation/1 -> Efficiency/1  "eta_22"
  2-D Lookup Table/1 -> Saturation/1
  Torque/1 -> Abs/1

== system TVModel_Simulation/Subsystem/Subsystem1/Torque Distribution/MPC/Weights generation/Subsystem1/Steer Activation/First Activation ==
  In1 : Inport
  AND1 : Logic  IconShape=distinctive  AllPortsSameDT=off  OutDataTypeStr=boolean
  Constant9 : Constant  Value=0
  Less Than3 : RelationalOperator  Operator===  OutDataTypeStr=boolean  RndMeth=Simplest  InputSameDT=off
  Less Than4 : RelationalOperator  Operator=<  OutDataTypeStr=boolean  RndMeth=Simplest  InputSameDT=off
  Unit Delay1 : UnitDelay  SampleTime=-1  HasFrameUpgradeWarning=on
  Out1 : Outport
  wires:
  Constant9/1 -> Less Than3/2, Less Than4/1
  Unit Delay1/1 -> Less Than3/1
  In1/1 -> Less Than4/2, Unit Delay1/1
  Less Than4/1 -> AND1/2
  Less Than3/1 -> AND1/1
  AND1/1 -> Out1/1

== system TVModel_Simulation/Subsystem/Subsystem1/Torque Distribution/MPC/Weights generation/Subsystem1/Steer Activation/If Action Subsystem ==
  Inport : Inport
  Action Port : ActionPort
  Data Type Conversion : DataTypeConversion  OutDataTypeStr=double  RndMeth=Nearest  SaturateOnIntegerOverflow=off
  Epsilon : Outport
  wires:
  Inport/1 -> Data Type Conversion/1
  Data Type Conversion/1 -> Epsilon/1

== system TVModel_Simulation/Subsystem/Subsystem1/Torque Distribution/MPC/Weights generation/Subsystem1/Steer Activation/If Action Subsystem1 ==
  Inport : Inport
  Action Port : ActionPort
  Constant : Constant  Value=1*pi/180
  Gain : Gain  Gain=1/(2*pi/180)
  Saturation : Saturate  UpperLimit=1  LowerLimit=0
  Saturation1 : Saturate  UpperLimit=inf  LowerLimit=0
  Subtract : Sum  Inputs=+-
  epsilon : Outport
  wires:
  Saturation1/1 -> Gain/1
  Saturation/1 -> epsilon/1
  Gain/1 -> Saturation/1
  Subtract/1 -> Saturation1/1
  Inport/1 -> Subtract/1
  Constant/1 -> Subtract/2

== matlab function TVModel_Simulation/Subsystem/Subsystem1/Torque Distribution/MPC/     Output vector reference/MATLAB Function ==
  data: vx input; vy_ref output; YRD input
function vy_ref = fcn(vx,YRD)

g   = 9.81;            % [m/s^2]                          
wd  = 0.5;             % [~]         
wb  = 1.53;            % [~]          
tf  = 1.27;            % [m]          
tr  = 1.27;            % [m]          
m   = 195+75;          % [Kg]            
Iz  = 120;             % [Kg*m^2]         
a   = wb*wd;           % [m]            
b   = wb - a;          % [m]            
hcog = 0.29;           % [m]           
Fzf  = m*g/2*(wd);     % [N]                 
Fzr  = m*g/2*(1-wd);   % [N]                   
tau = 13.5;            % [~]          
rs  = 0.235;           % [m] 

Cr = 60*10^3;
% K = -1e-03;

% YRD = vx.*(delta./(wb.*1+K.*vx.^2));
beta_ref = (b./vx - m.*a.*vx./wb/Cr).*YRD;

vy_ref = -vx.*tan(beta_ref);
vy_ref = 0;

== matlab function TVModel_Simulation/Subsystem/Subsystem1/Torque Distribution/MPC/     Output vector reference/MATLAB Function1 ==
  data: vx input; vx_ref output; vy input; acc input
function vx_ref = fcn(vx,vy,acc)

g   = 9.81;            % [m/s^2]                          
wd  = 0.5;             % [~]         
wb  = 1.53;            % [~]          
tf  = 1.27;            % [m]          
tr  = 1.27;            % [m]          
m   = 195+75;          % [Kg]            
Iz  = 120;             % [Kg*m^2]         
a   = wb*wd;           % [m]            
b   = wb - a;          % [m]            
hcog = 0.29;           % [m]           
Fzf  = m*g/2*(wd);     % [N]                 
Fzr  = m*g/2*(1-wd);   % [N]                   
tau = 13.5;            % [~]          
rs  = 0.235;           % [m] 

Mt = acc*4*20;
vx_ref = sqrt(vx^2+vy^2) + tau/rs*Mt*10*0.02/220;
vx_ref = 0;

== matlab function TVModel_Simulation/Subsystem/Subsystem1/Torque Distribution/MPC/ States/Extended Kalman Filter/measurement_kalman_simulink/h(x) ==
  data: x input; y output
function y = measurement_kalman_simulink(x)

y = zeros(3,1);
y(1) = x(1);
y(2) = x(2);
y(3) = x(3);

end
